simulink model "sim_6_dof"  (R2019b)
settings: Solver=ode4  StartTime=0.0  StopTime=tf  FixedStep=dt  RelTol=1e-3
values from neighbouring files (symbols this model uses):
  F = [ F_X ; F_Y ; F_Z ]    [get_states_dot.m]
undefined symbols (not defined in the file or in its folder): epsi_0, M, p_0, phi_0, q_0, r_0, theta_0, u_0, v_0, w_0, x_0, y_0, z_0
libraries: shared6dof x1
settings Model: Creator=yossef  LastModifiedBy=Yousef
settings DataIOCC: ReturnWorkspaceOutputs=off
settings DebuggingCC: ArithmeticOperatorsInVariantConditions=warning
settings SFSimCC: SimUseLocalCustomCode=off  CustomCodeUndefinedFunction=UseInterfaceOnly
settings RTWCC: RTWUseLocalCustomCode=off

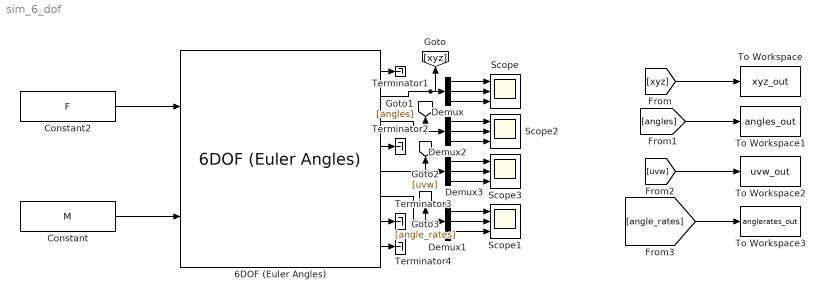
== system sim_6_dof ==
  6DOF (Euler Angles) : shared6dof/6DOF (Euler Angles)  units=Metric (MKS)  mtype=Fixed  rep=Euler Angles  xme_0=[x_0 y_0 z_0]  Vm_0=[u_0 v_0 w_0]  eul_0=[phi_0 theta_0 epsi_0]  pm_0=[p_0 q_0 r_0]  mass_0=m  mass_e=0.5  mass_f=2.0  inertia=I  inertia_e=eye(3)  inertia_f=2*eye(3)  k_quat=1.0  vre_flag=on  abi_flag=off  aMode=0  xme_statename=''  Vm_statename=''  eul_statename=''  quat_statename=''  pm_statename=''  mass_statename=''
      settings: SourceProductBaseCode=AE
  Constant : Constant  Value=M
  Constant2 : Constant  Value=F
  Demux{,1..3} (4 alike) : Demux  Outputs=3
  Scope{,1..3} (4 alike) : Scope  NumInputPorts=3
  Terminator{1..4} (4 alike) : Terminator
  To Workspace : ToWorkspace  VariableName=xyz_out  SampleTime=-1
  To Workspace1 : ToWorkspace  VariableName=angles_out  SampleTime=-1
  To Workspace2 : ToWorkspace  VariableName=uvw_out  SampleTime=-1
  To Workspace3 : ToWorkspace  VariableName=anglerates_out  SampleTime=-1
  wires:
  Constant2/1 -> 6DOF (Euler Angles)/1
  Constant/1 -> 6DOF (Euler Angles)/2
  6DOF (Euler Angles)/1 -> Terminator1/1
  6DOF (Euler Angles)/2 -> Demux/1, [xyz]
  6DOF (Euler Angles)/6 -> [angle_rates], Demux1/1
  Demux/1 -> Scope/1
  Demux/2 -> Scope/2
  Demux/3 -> Scope/3
  6DOF (Euler Angles)/3 -> Demux2/1, [angles]
  Demux2/1 -> Scope2/1
  Demux2/2 -> Scope2/2
  Demux2/3 -> Scope2/3
  6DOF (Euler Angles)/4 -> Terminator2/1
  Demux3/1 -> Scope3/1
  Demux3/2 -> Scope3/2
  Demux3/3 -> Scope3/3
  6DOF (Euler Angles)/5 -> [uvw], Demux3/1
  6DOF (Euler Angles)/7 -> Terminator3/1
  6DOF (Euler Angles)/8 -> Terminator4/1
  Demux1/1 -> Scope1/1
  Demux1/2 -> Scope1/2
  Demux1/3 -> Scope1/3
  [xyz] -> To Workspace/1
  [angles] -> To Workspace1/1
  [uvw] -> To Workspace2/1
  [angle_rates] -> To Workspace3/1
